simulink model "Forward_model_V4"  (R2018a)
settings: Solver=ode1  StartTime=0.0  StopTime=30  FixedStep=0.001  RelTol=1e-3
InitFcn:
  | Main
values from neighbouring files (symbols this model uses):
  tra_01 = tra_01'    [tra.m]
  tra_02 = tra_02'    [tra.m]
  tra_03 = tra_03'    [tra.m]
  tra_04 = tra_04'    [tra.m]
  tra_05 = tra_05'    [tra.m]
  tra_06 = tra_06'    [tra.m]
undefined symbols (not defined in the file or in its folder): DiscIntNeverNeededParam
libraries: simulink x2
settings Model: Creator=yuxi  LastModifiedBy=yuxi
settings SolverCC: AlgebraicLoopSolver=LineSearch

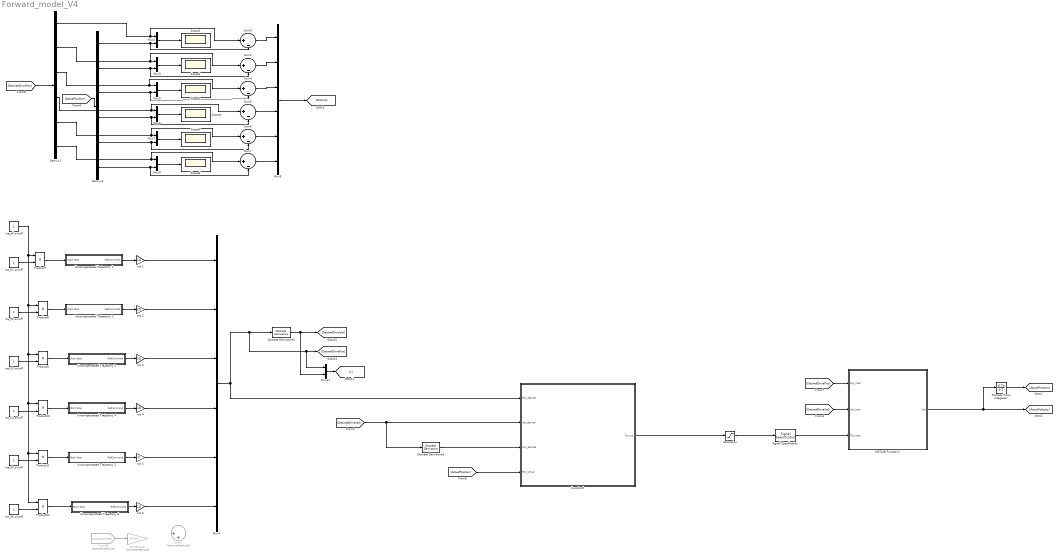
== system Forward_model_V4 ==
  " Function5" : MATLAB Function  TreatAsAtomicUnit=on
  Act J6 pos2 : Gain  Commented=on  Gain=0.025
  Demux1 : Demux  Outputs=6
  Demux4 : Demux  Outputs=6
  Discrete Derivative2 : simulink/Discrete/Discrete Derivative  gainval=1.0  ICPrevScaledInput=0.0  InputProcessing=Inherited  OutMin=[]  OutMax=[]  OutDataType=fixdt(1, 16)  OutScaling=2^-10  DoSatur=off
  Discrete Derivative3 : simulink/Discrete/Discrete Derivative  gainval=1.0  ICPrevScaledInput=0.0  InputProcessing=Inherited  OutMin=[]  OutMax=[]  OutDataType=fixdt(1, 16)  OutScaling=2^-10  DoSatur=off
  Discrete-Time Integrator : DiscreteIntegrator  SampleTime=-1  ICPrevOutput=DiscIntNeverNeededParam  ICPrevScaledInput=DiscIntNeverNeededParam
  From31 : From  Commented=on  GotoTag=ActualPosition5
  MATLAB Function2 : MATLAB Function  TreatAsAtomicUnit=on
  Mux{2..3,5..8,11} (7 alike) : Mux  Inputs=2
  Mux4 : Mux  Inputs=6
  Mux9 : Mux  Inputs=6
  Product{7..12} (6 alike) : Product  RndMeth=Zero
  Saturation : Saturate  UpperLimit=6  LowerLimit=-6
  Scope{1..6} (6 alike) : Scope
  Signal Specification : SignalSpecification  Dimensions=6
  Sum1 : Sum  Commented=on  Inputs=|++
  Sum{2..7} (6 alike) : Sum  Inputs=|+-
  Uncompensated Trajectory 1 : Subsystem
  Uncompensated Trajectory 2 : Subsystem
  Uncompensated Trajectory 3 : Subsystem
  Uncompensated Trajectory 4 : Subsystem
  Uncompensated Trajectory 5 : Subsystem
  Uncompensated Trajectory 6 : Subsystem
  tra 1 : Gain  Gain=10
  tra 2 : Gain  Gain=10
  "tra 3 " : Gain  Gain=10
  "tra 4 " : Gain  Gain=10
  "tra 5 " : Gain  Gain=0
  "tra 6 " : Gain  Gain=10
  tra_01 on/off : Constant
  tra_02 on/off : Constant
  tra_03 on/off : Constant
  tra_04 on/off : Constant
  tra_05 on/off : Constant
  tra_06 on/off : Constant
  tra_all on/off : Constant
  wires:
  [DesiredDrivePos] -> Demux1/1
  [ActualPosition] -> Demux4/1
  Uncompensated Trajectory 2/1(RefCommand) -> tra 2/1
  Uncompensated Trajectory 4/1(RefCommand) -> "tra 4 "/1
  tra_06 on/off/1 -> Product12/2
  Uncompensated Trajectory 1/1(RefCommand) -> tra 1/1
  From31/1 -> Act J6 pos2/1
  tra_02 on/off/1 -> Product8/2
  Product12/1 -> Uncompensated Trajectory 6/1(Start-Stop)
  Product9/1 -> Uncompensated Trajectory 3/1(Start-Stop)
  tra_03 on/off/1 -> Product9/2
  Product11/1 -> Uncompensated Trajectory 5/1(Start-Stop)
  Product10/1 -> Uncompensated Trajectory 4/1(Start-Stop)
  Product7/1 -> Uncompensated Trajectory 1/1(Start-Stop)
  Uncompensated Trajectory 3/1(RefCommand) -> "tra 3 "/1
  tra_04 on/off/1 -> Product10/2
  Uncompensated Trajectory 5/1(RefCommand) -> "tra 5 "/1
  tra_05 on/off/1 -> Product11/2
  Product8/1 -> Uncompensated Trajectory 2/1(Start-Stop)
  Uncompensated Trajectory 6/1(RefCommand) -> "tra 6 "/1
  tra_all on/off/1 -> Product9/1, Product10/1, Product11/1, Product12/1, Product8/1, Product7/1
  tra_01 on/off/1 -> Product7/2
  Discrete-Time Integrator/1 -> [ActualPosition]
  [DesiredDrivePos] -> MATLAB Function2/1(Pos_input)
  [DesiredDriveVel] -> MATLAB Function2/2(Vel_input)
  Demux4/1 -> Sum3/2, Mux2/2
  Demux1/1 -> Sum3/1, Mux2/1
  Demux4/2 -> Sum2/2, Mux3/2
  Demux1/2 -> Sum2/1, Mux3/1
  Demux4/4 -> Sum5/2, Mux6/2
  Demux1/4 -> Sum5/1, Mux6/1
  Demux4/5 -> Sum6/2, Mux7/2
  Demux1/5 -> Sum6/1, Mux7/1
  Demux4/6 -> Sum7/2, Mux8/2
  Demux1/6 -> Sum7/1, Mux8/1
  tra 1/1 -> Mux4/1
  tra 2/1 -> Mux4/2
  "tra 3 "/1 -> Mux4/3
  "tra 4 "/1 -> Mux4/4
  "tra 5 "/1 -> Mux4/5
  "tra 6 "/1 -> Mux4/6
  Mux2/1 -> Scope1/1
  Mux3/1 -> Scope2/1
  Mux5/1 -> Scope3/1
  Mux6/1 -> Scope4/1
  Mux7/1 -> Scope5/1
  Mux8/1 -> Scope6/1
  [DesiredDriveVel] -> Discrete Derivative3/1, " Function5"/2(Vel_desired)
  Discrete Derivative3/1 -> " Function5"/3(Acc_desired)
  Demux1/3 -> Sum4/1, Mux5/1
  Demux4/3 -> Sum4/2, Mux5/2
  Sum6/1 -> Mux9/5
  Sum7/1 -> Mux9/6
  Sum4/1 -> Mux9/3
  Sum2/1 -> Mux9/2
  Sum3/1 -> Mux9/1
  Mux9/1 -> [Disturb]
  Sum5/1 -> Mux9/4
  MATLAB Function2/1(Vel) -> [ActualVelosity], Discrete-Time Integrator/1
  Saturation/1 -> Signal Specification/1
  Signal Specification/1 -> MATLAB Function2/3(Tor_input)
  Mux4/1 -> [DesiredDrivePos], Mux11/1, Discrete Derivative2/1, " Function5"/1(Pos_desired)
  Discrete Derivative2/1 -> [DesiredDriveVel], Mux11/2
  Mux11/1 -> [y]
  " Function5"/1(Tor_out) -> Saturation/1
  [ActualPosition] -> " Function5"/4(Pos_Actual)

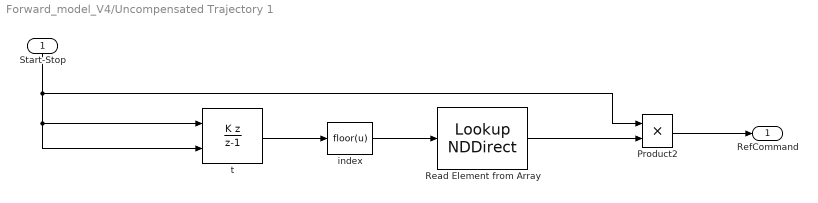
== system Forward_model_V4/Uncompensated Trajectory 1 ==
  Start-Stop : Inport
  Product2 : Product  RndMeth=Zero
  Read Element from Array : LookupNDDirect  NumberOfTableDimensions=1  Table=tra_01
  index : Fcn  Expr=floor(u)
  t : DiscreteIntegrator  IntegratorMethod=Accumulation: Backward Euler  ExternalReset=rising  SampleTime=-1  ICPrevOutput=DiscIntNeverNeededParam  ICPrevScaledInput=DiscIntNeverNeededParam
  RefCommand : Outport
  wires:
  Read Element from Array/1 -> Product2/2
  t/1 -> index/1
  Product2/1 -> RefCommand/1
  Start-Stop/1 -> Product2/1, t/1, t/2
  index/1 -> Read Element from Array/1

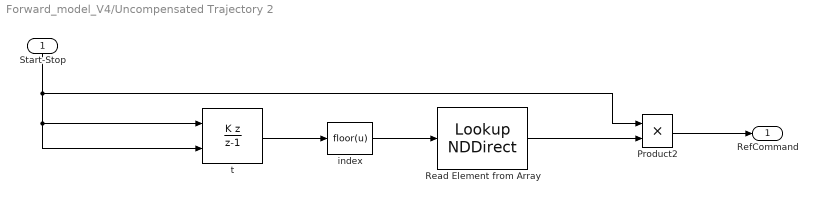
== system Forward_model_V4/Uncompensated Trajectory 2 ==
  Start-Stop : Inport
  Product2 : Product  RndMeth=Zero
  Read Element from Array : LookupNDDirect  NumberOfTableDimensions=1  Table=tra_02
  index : Fcn  Expr=floor(u)
  t : DiscreteIntegrator  IntegratorMethod=Accumulation: Backward Euler  ExternalReset=rising  SampleTime=-1  ICPrevOutput=DiscIntNeverNeededParam  ICPrevScaledInput=DiscIntNeverNeededParam
  RefCommand : Outport
  wires:
  index/1 -> Read Element from Array/1
  Start-Stop/1 -> t/2, t/1, Product2/1
  Product2/1 -> RefCommand/1
  t/1 -> index/1
  Read Element from Array/1 -> Product2/2

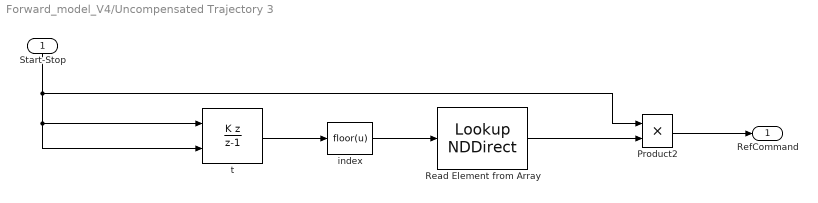
== system Forward_model_V4/Uncompensated Trajectory 3 ==
  Start-Stop : Inport
  Product2 : Product  RndMeth=Zero
  Read Element from Array : LookupNDDirect  NumberOfTableDimensions=1  Table=tra_03
  index : Fcn  Expr=floor(u)
  t : DiscreteIntegrator  IntegratorMethod=Accumulation: Backward Euler  ExternalReset=rising  SampleTime=-1  ICPrevOutput=DiscIntNeverNeededParam  ICPrevScaledInput=DiscIntNeverNeededParam
  RefCommand : Outport
  wires:
  Read Element from Array/1 -> Product2/2
  t/1 -> index/1
  Product2/1 -> RefCommand/1
  Start-Stop/1 -> Product2/1, t/1, t/2
  index/1 -> Read Element from Array/1

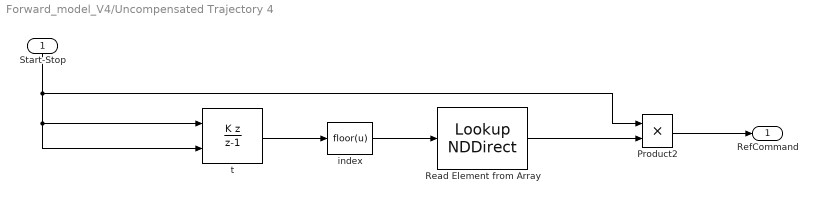
== system Forward_model_V4/Uncompensated Trajectory 4 ==
  Start-Stop : Inport
  Product2 : Product  RndMeth=Zero
  Read Element from Array : LookupNDDirect  NumberOfTableDimensions=1  Table=tra_04
  index : Fcn  Expr=floor(u)
  t : DiscreteIntegrator  IntegratorMethod=Accumulation: Backward Euler  ExternalReset=rising  SampleTime=-1  ICPrevOutput=DiscIntNeverNeededParam  ICPrevScaledInput=DiscIntNeverNeededParam
  RefCommand : Outport
  wires:
  Read Element from Array/1 -> Product2/2
  t/1 -> index/1
  Product2/1 -> RefCommand/1
  Start-Stop/1 -> Product2/1, t/1, t/2
  index/1 -> Read Element from Array/1

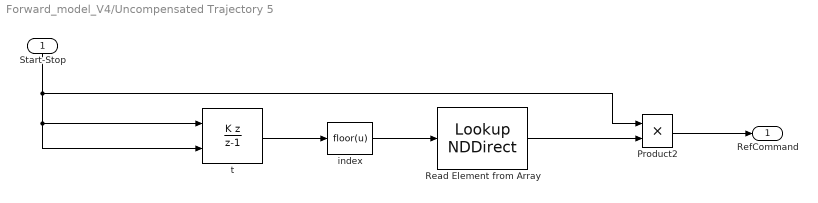
== system Forward_model_V4/Uncompensated Trajectory 5 ==
  Start-Stop : Inport
  Product2 : Product  RndMeth=Zero
  Read Element from Array : LookupNDDirect  NumberOfTableDimensions=1  Table=tra_05
  index : Fcn  Expr=floor(u)
  t : DiscreteIntegrator  IntegratorMethod=Accumulation: Backward Euler  ExternalReset=rising  SampleTime=-1  ICPrevOutput=DiscIntNeverNeededParam  ICPrevScaledInput=DiscIntNeverNeededParam
  RefCommand : Outport
  wires:
  Read Element from Array/1 -> Product2/2
  t/1 -> index/1
  Product2/1 -> RefCommand/1
  Start-Stop/1 -> Product2/1, t/1, t/2
  index/1 -> Read Element from Array/1

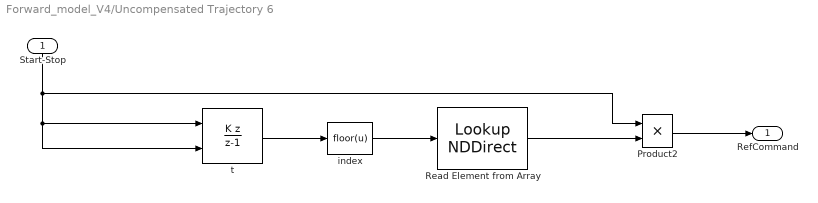
== system Forward_model_V4/Uncompensated Trajectory 6 ==
  Start-Stop : Inport
  Product2 : Product  RndMeth=Zero
  Read Element from Array : LookupNDDirect  NumberOfTableDimensions=1  Table=tra_06
  index : Fcn  Expr=floor(u)
  t : DiscreteIntegrator  IntegratorMethod=Accumulation: Backward Euler  ExternalReset=rising  SampleTime=-1  ICPrevOutput=DiscIntNeverNeededParam  ICPrevScaledInput=DiscIntNeverNeededParam
  RefCommand : Outport
  wires:
  index/1 -> Read Element from Array/1
  Start-Stop/1 -> t/2, t/1, Product2/1
  Product2/1 -> RefCommand/1
  t/1 -> index/1
  Read Element from Array/1 -> Product2/2

== matlab function Forward_model_V4/MATLAB Function2 ==
  data: Pos_input input; Vel_input input; Tor_input input; Vel output; Ts parameter
% Input -- jnt_val: 3x6 -> Joint angles, velocities and accelerations of 6 actuated joints
% [
%   ang_1, ang_2, ang_3, ang_4, ang_5, ang_6;
%   vel_1, vel_2, vel_3, vel_4, vel_5, vel_6;
%   acc_1, acc_2, acc_3, acc_4, acc_5, acc_6;
% ]
% Output -- torques: 6x1 -> For 6 joints
% Time required: 0.25ms
% function [Pos, Vel, Acc] = Robot(ActualPos, ActualVel, Tor)

% This is the forward model of Julun robot, it can be used in simulation
% The author is YuXi

% Pos_input = rand(1,6);
% Vel_input = rand(1,6);
% ActualAcc = zeros(1,6);
% Tor_input = rand(6,1);


function Vel = Robot_model(Pos_input, Vel_input, Tor_input, Ts)

% download the position commands of each joint
Pos_joint1 = Pos_input(1);
Pos_joint2 = Pos_input(2);
Pos_joint3 = Pos_input(3);
Pos_joint4 = Pos_input(4);
Pos_joint5 = Pos_input(5);
Pos_joint6 = Pos_input(6);
Pos_commands = [Pos_joint1 Pos_joint2 Pos_joint3 Pos_joint4 Pos_joint5 Pos_joint6];

% download the velocity commands of each joint
Vel_joint1 = Vel_input(1);
Vel_joint2 = Vel_input(2);
Vel_joint3 = Vel_input(3);
Vel_joint4 = Vel_input(4);
Vel_joint5 = Vel_input(5);
Vel_joint6 = Vel_input(6);
Vel_commands = [Vel_joint1 Vel_joint2 Vel_joint3 Vel_joint4 Vel_joint5 Vel_joint6];

% downlaod the torque informations of each joint
Tor_joint1 = Tor_input(1);
Tor_joint2 = Tor_input(2);
Tor_joint3 = Tor_input(3);
Tor_joint4 = Tor_input(4);
Tor_joint5 = Tor_input(5);
Tor_joint6 = Tor_input(6);
Tor = [Tor_joint1 Tor_joint2 Tor_joint3 Tor_joint4 Tor_joint5 Tor_joint6]';

%% compute the Cdq+Gq

DH = [0, 0, 0, 0; 0, 0.19, pi/2, pi/2; 0, 0.65, 0, 0; 0.73, 0.192, pi/2, 0; 0, 0, pi/2, 0; 0, 0, -pi/2, 0];
iVector = [0,0,0,0,0.844903,0;-0.324345,-0.075914,-0.051391,-0.042523,0.740601,0;-0.091039,0.053809,0.006962,-0.031913,0.049886,0;-0.009236,-0.006692,-0.011727,-0.000768,0.020729,0;-0.004762,0.002377,-0.001658,0.003359,0.000719,0;-0.005854,-0.004165,-0.005599,0.002253,0.001373,0];
mCenter = [0,0.327776,0.067582,-0.004515,0.003987,0.000929;0,0.021804,-0.089291,0.002001,0.00702,-0.001923;0,0,0,0,0,0];
Ia = [0.259947,-0.014791,0.040481,0.013916];
% Fs = [0.372305,0.494409,0.409654,0.063411,0.32759,0.197599];
% Fv = [1.610821,1.074123,0.624158,0.264797,0.327863,0.311985];
% Ia = [0 0 0 0];
Fs = [0 0 0 0 0 0];
Fv = [0 0 0 0 0 0];

iMatrix=zeros(3,3,6);
for i = 1 : 6
    iMatrix(:, :, i) = [iVector(i, 1), iVector(i, 2), iVector(i, 3); iVector(i, 2), iVector(i, 6), iVector(i, 4); iVector(i, 3), iVector(i, 4), iVector(i, 5)];
end   
    
acc_defined = zeros(1,6);       % Set the acceleration to 0, and then compute the torque_*
tor = zeros(6, 1);
rot=zeros(3,3,6);
omega=zeros(3,6);
domega=zeros(3,6);
accer=zeros(3,6);
cforce=zeros(3,6);
force=zeros(3,6);
torque=zeros(3,6);

qval = Pos_commands(1, :);
dqval = Vel_commands(1, :);
ddqval = acc_defined(1, :);
theta = DH(:, 4)' + qval;
pos = [DH(:, 2)'; -(DH(:, 1).*sin(DH(:, 3)))'; (DH(:, 1).*cos(DH(:, 3)))'];

for i = 1 : 6
    rot(:, :, i) = [cos(theta(i)), cos(DH(i, 3))*sin(theta(i)), sin(DH(i, 3))*sin(theta(i)); -sin(theta(i)), cos(DH(i, 3))*cos(theta(i)), sin(DH(i, 3))*cos(theta(i)); 0, -sin(DH(i, 3)), cos(DH(i, 3))];
end

i = 0;
omega_0 = zeros(3, 1);
domega_0 = zeros(3, 1);
accer_0 = [0; 0; 9.80665];
i = 1;
omega(:, i) = [0; 0; dqval(i)];
domega(:, i) = [0; 0; ddqval(i)];
accer(:, i) = rot(:, :, i) * accer_0;
cforce(:, i) = cross(domega(:, i), mCenter(:, i)) + cross(omega(:, i), cross(omega(:, i), mCenter(:, i)));

for i = 2 : 6
    omega(:, i) = rot(:, :, i) * omega(:, i - 1) + [0; 0; dqval(i)];
    domega(:, i) = rot(:, :, i) * domega(:, i - 1) + cross(rot(:, :, i)*omega(:, i - 1), [0; 0; dqval(i)]) + [0; 0; ddqval(i)];
    accer(:, i) = rot(:, :, i) * (accer(:, i - 1) + (cross(domega(:, i - 1), pos(:, i))) + (cross(omega(:, i - 1), cross(omega(:, i - 1), pos(:, i)))));
    cforce(:, i) = cross(domega(:, i), mCenter(:, i)) + cross(omega(:, i), cross(omega(:, i), mCenter(:, i)));
end

i = 6;
force(:, i) = cforce(:, i);
torque(:, i) = iMatrix(:, :, i) * domega(:, i) + cross(omega(:, i), iMatrix(:, :, i)*omega(:, i)) + cross(mCenter(:, i), accer(:, i));
tor(i) = torque(3, i);

for i = 5 : -1 : 1
    force(:, i) = cforce(:, i) + rot(:, :, i+1)' * force(:, i+1);
    torque(:, i) = iMatrix(:, :, i) * domega(:, i) + cross(omega(:, i), iMatrix(:, :, i)*omega(:, i)) + cross(mCenter(:, i), accer(:, i)) + rot(:, :, i+1)' * torque(:, i+1) + cross(pos(:, i+1), rot(:, :, i+1)'*force(:, i+1));
    tor(i) = torque(3, i);
end

tor = tor + (Fs.*sign(dqval))' + (Fv.*dqval)' + ([0, 0, Ia].*ddqval)';

% tor = tor + ([0, 0, Ia].*ddqval)';
Tor_delta = Tor - tor;

%% compute the M(q)

Eye_matrix = eye(6);
tor = zeros(6, 1);
rot=zeros(3,3,6);
omega=zeros(3,6);
domega=zeros(3,6);
accer=zeros(3,6);
cforce=zeros(3,6);
force=zeros(3,6);
torque=zeros(3,6);
H = zeros(6,6);
Vel_commands2 = zeros(1,6);                % Set the velocity to 0

for j = 1:6
    acc_defined2 = Eye_matrix(:,j)';       % Set each colume to unit vector
    qval = Pos_commands(1, :);
    dqval = Vel_commands2(1, :);
    ddqval = acc_defined2(1, :);
    theta = DH(:, 4)' + qval;
    pos = [DH(:, 2)'; -(DH(:, 1).*sin(DH(:, 3)))'; (DH(:, 1).*cos(DH(:, 3)))'];
    
    for i = 1 : 6
        rot(:, :, i) = [cos(theta(i)), cos(DH(i, 3))*sin(theta(i)), sin(DH(i, 3))*sin(theta(i)); -sin(theta(i)), cos(DH(i, 3))*cos(theta(i)), sin(DH(i, 3))*cos(theta(i)); 0, -sin(DH(i, 3)), cos(DH(i, 3))];
    end
    
    i = 0;
    omega_0 = zeros(3, 1);
    domega_0 = zeros(3, 1);
    accer_0 = [0; 0; 0];        % 重力加速度设置为0
    i = 1;
    omega(:, i) = [0; 0; dqval(i)];
    domega(:, i) = [0; 0; ddqval(i)];
    accer(:, i) = rot(:, :, i) * accer_0;
    cforce(:, i) = cross(domega(:, i), mCenter(:, i)) + cross(omega(:, i), cross(omega(:, i), mCenter(:, i)));
    cforce(:, i) = cross(domega(:, i), mCenter(:, i)) + cross(omega(:, i), cross(omega(:, i), mCenter(:, i)));
    
    for i = 2 : 6
        omega(:, i) = rot(:, :, i) * omega(:, i - 1) + [0; 0; dqval(i)];
        domega(:, i) = rot(:, :, i) * domega(:, i - 1) + cross(rot(:, :, i)*omega(:, i - 1), [0; 0; dqval(i)]) + [0; 0; ddqval(i)];
        accer(:, i) = rot(:, :, i) * (accer(:, i - 1) + (cross(domega(:, i - 1), pos(:, i))) + (cross(omega(:, i - 1), cross(omega(:, i - 1), pos(:, i)))));
        cforce(:, i) = cross(domega(:, i), mCenter(:, i)) + cross(omega(:, i), cross(omega(:, i), mCenter(:, i)));
    end
    
    i = 6;
    force(:, i) = cforce(:, i);
    torque(:, i) = iMatrix(:, :, i) * domega(:, i) + cross(omega(:, i), iMatrix(:, :, i)*omega(:, i)) + cross(mCenter(:, i), accer(:, i));
    tor(i) = torque(3, i);
    
    for i = 5 : -1 : 1
        force(:, i) = cforce(:, i) + rot(:, :, i+1)' * force(:, i+1);
        torque(:, i) = iMatrix(:, :, i) * domega(:, i) + cross(omega(:, i), iMatrix(:, :, i)*omega(:, i)) + cross(mCenter(:, i), accer(:, i)) + rot(:, :, i+1)' * torque(:, i+1) + cross(pos(:, i+1), rot(:, :, i+1)'*force(:, i+1));
        tor(i) = torque(3, i);
    end
    
%     H(:,j) = tor + (Fs.*sign(dqval))' + (Fv.*dqval)';
    H(:,j) = tor;
    
end

%% compute the ddq

% Acc = (inv(H) * Tor_delta)';
Acc = (inv(H + diag([0, 0, Ia])) * Tor_delta)';
Vel = (Vel_commands + Acc * Ts)';

% Pos = (Pos_commands + Vel_commands * Ts + 0.5 * Acc * (Ts).^2)';    
          
end

== matlab function Forward_model_V4/ Function5 ==
  data: Tor_out output; Pos_desired input; Vel_desired input; Acc_desired input; Pos_Actual input

% function Vel = Robot_LQR(Pos_input, Vel_input, Tor_input, Ts)

% Input -- jnt_val: 3x6 -> Joint angles, velocities and accelerations of 6 actuated joints
% [
%   ang_1, ang_2, ang_3, ang_4, ang_5, ang_6;
%   vel_1, vel_2, vel_3, vel_4, vel_5, vel_6;
%   acc_1, acc_2, acc_3, acc_4, acc_5, acc_6;
% ]
% Output -- torques: 6x1 -> For 6 joints
% Time required: 0.25ms
% function [Pos, Vel, Acc] = Robot(ActualPos, ActualVel, Tor)

% This is the forward model of Julun robot, it can be used in simulation
% The author is YuXi

% function [Tor_out, A, B, H, D] = Robot_LQR_X(Pos_desired, Vel_desired, Acc_desired, Actual_Esti)
function Tor_out  = Robot_LQR_X(Pos_desired, Vel_desired, Acc_desired, Pos_Actual)


% Pos_desired = rand(1,6);
% Pos_actual = Pos_desired;
% Vel_desired = rand(1,6);
% Vel_actual = Vel_desired;
% Acc_actual = rand(1,6);

coder.extrinsic('lqr');

% download the desired position commands of each joint
Pos_j1 = Pos_desired(1);
Pos_j2 = Pos_desired(2);
Pos_j3 = Pos_desired(3);
Pos_j4 = Pos_desired(4);
Pos_j5 = Pos_desired(5);
Pos_j6 = Pos_desired(6);
Pos_Desired = [Pos_j1 Pos_j2 Pos_j3 Pos_j4 Pos_j5 Pos_j6];
% Pos_Desired = [Pos_j1 Pos_j2 Pos_j3 Pos_j4 Pos_j5 Pos_j6 zeros(1,6)];

% download the desired position commands of each joint
Vel_j1 = Vel_desired(1);
Vel_j2 = Vel_desired(2);
Vel_j3 = Vel_desired(3);
Vel_j4 = Vel_desired(4);
Vel_j5 = Vel_desired(5);
Vel_j6 = Vel_desired(6);
Vel_Desired = [Vel_j1 Vel_j2 Vel_j3 Vel_j4 Vel_j5 Vel_j6];

% download the actual acceleration commands of each joint
Acc_joint1 = Acc_desired(1);
Acc_joint2 = Acc_desired(2);
Acc_joint3 = Acc_desired(3);
Acc_joint4 = Acc_desired(4);
Acc_joint5 = Acc_desired(5);
Acc_joint6 = Acc_desired(6);
Acc_Desired = [Acc_joint1 Acc_joint2 Acc_joint3 Acc_joint4 Acc_joint5 Acc_joint6];

%% the parameters

DH = [0, 0, 0, 0; 0, 0.19, pi/2, pi/2; 0, 0.65, 0, 0; 0.73, 0.192, pi/2, 0; 0, 0, pi/2, 0; 0, 0, -pi/2, 0];
iVector = [0,0,0,0,0.844903,0;-0.324345,-0.075914,-0.051391,-0.042523,0.740601,0;-0.091039,0.053809,0.006962,-0.031913,0.049886,0;-0.009236,-0.006692,-0.011727,-0.000768,0.020729,0;-0.004762,0.002377,-0.001658,0.003359,0.000719,0;-0.005854,-0.004165,-0.005599,0.002253,0.001373,0];
mCenter = [0,0.327776,0.067582,-0.004515,0.003987,0.000929;0,0.021804,-0.089291,0.002001,0.00702,-0.001923;0,0,0,0,0,0];
Ia = [0.259947,-0.014791,0.040481,0.013916];
% Fs = [0.372305,0.494409,0.409654,0.063411,0.32759,0.197599];
% Fv = [1.610821,1.074123,0.624158,0.264797,0.327863,0.311985];
% Ia = [0 0 0 0];
Fs = [0 0 0 0 0 0];
Fv = [0 0 0 0 0 0];

iMatrix=zeros(3,3,6);
for i = 1 : 6
    iMatrix(:, :, i) = [iVector(i, 1), iVector(i, 2), iVector(i, 3); iVector(i, 2), iVector(i, 6), iVector(i, 4); iVector(i, 3), iVector(i, 4), iVector(i, 5)];
end

%% the Tor_all

tor = zeros(6, 1);
rot=zeros(3,3,6);
omega=zeros(3,6);
domega=zeros(3,6);
accer=zeros(3,6);
cforce=zeros(3,6);
force=zeros(3,6);
torque=zeros(3,6);

qval = Pos_Desired(1, :);
dqval = Vel_Desired(1, :);
ddqval = Acc_Desired(1, :);
theta = DH(:, 4)' + qval;
pos = [DH(:, 2)'; -(DH(:, 1).*sin(DH(:, 3)))'; (DH(:, 1).*cos(DH(:, 3)))'];
for i = 1 : 6
    rot(:, :, i) = [cos(theta(i)), cos(DH(i, 3))*sin(theta(i)), sin(DH(i, 3))*sin(theta(i)); -sin(theta(i)), cos(DH(i, 3))*cos(theta(i)), sin(DH(i, 3))*cos(theta(i)); 0, -sin(DH(i, 3)), cos(DH(i, 3))];
end
i = 0;
omega_0 = zeros(3, 1);
domega_0 = zeros(3, 1);
accer_0 = [0; 0; 9.80665];
i = 1;
omega(:, i) = [0; 0; dqval(i)];
domega(:, i) = [0; 0; ddqval(i)];
accer(:, i) = rot(:, :, i) * accer_0;
cforce(:, i) = cross(domega(:, i), mCenter(:, i)) + cross(omega(:, i), cross(omega(:, i), mCenter(:, i)));
for i = 2 : 6
    omega(:, i) = rot(:, :, i) * omega(:, i - 1) + [0; 0; dqval(i)];
    domega(:, i) = rot(:, :, i) * domega(:, i - 1) + cross(rot(:, :, i)*omega(:, i - 1), [0; 0; dqval(i)]) + [0; 0; ddqval(i)];
    accer(:, i) = rot(:, :, i) * (accer(:, i - 1) + (cross(domega(:, i - 1), pos(:, i))) + (cross(omega(:, i - 1), cross(omega(:, i - 1), pos(:, i)))));
    cforce(:, i) = cross(domega(:, i), mCenter(:, i)) + cross(omega(:, i), cross(omega(:, i), mCenter(:, i)));
end
i = 6;
force(:, i) = cforce(:, i);
torque(:, i) = iMatrix(:, :, i) * domega(:, i) + cross(omega(:, i), iMatrix(:, :, i)*omega(:, i)) + cross(mCenter(:, i), accer(:, i));
tor(i) = torque(3, i);
for i = 5 : -1 : 1
    force(:, i) = cforce(:, i) + rot(:, :, i+1)' * force(:, i+1);
    torque(:, i) = iMatrix(:, :, i) * domega(:, i) + cross(omega(:, i), iMatrix(:, :, i)*omega(:, i)) + cross(mCenter(:, i), accer(:, i)) + rot(:, :, i+1)' * torque(:, i+1) + cross(pos(:, i+1), rot(:, :, i+1)'*force(:, i+1));
    tor(i) = torque(3, i);
end
Tor = tor;
Tor_d = (Fs.*sign(Vel_Desired))' + (Fv.*Vel_Desired)'  + ([0, 0, Ia].*ddqval)';
% Tor_d = (Fv.*Vel_Desired)'  + ([0, 0, Ia].*ddqval)';

%% compute the Hq.  The matrix of M(q)

Eye_matrix = eye(6);
tor = zeros(6, 1);
rot=zeros(3,3,6);
omega=zeros(3,6);
domega=zeros(3,6);
accer=zeros(3,6);
cforce=zeros(3,6);
force=zeros(3,6);
torque=zeros(3,6);
M = zeros(6,6);
Vel_commands2 = zeros(1,6);                % Set the velocity to 0    

for j = 1:6
    acc_defined2 = Eye_matrix(:,j)';       % Set each colume to unit vector
    qval = Pos_Desired(1, :);
    dqval = Vel_commands2(1, :);
    ddqval = acc_defined2(1, :);
    theta = DH(:, 4)' + qval;
    pos = [DH(:, 2)'; -(DH(:, 1).*sin(DH(:, 3)))'; (DH(:, 1).*cos(DH(:, 3)))'];
    
    for i = 1 : 6
        rot(:, :, i) = [cos(theta(i)), cos(DH(i, 3))*sin(theta(i)), sin(DH(i, 3))*sin(theta(i)); -sin(theta(i)), cos(DH(i, 3))*cos(theta(i)), sin(DH(i, 3))*cos(theta(i)); 0, -sin(DH(i, 3)), cos(DH(i, 3))];
    end
    
    i = 0;
    omega_0 = zeros(3, 1);
    domega_0 = zeros(3, 1);
    accer_0 = [0; 0; 0];        % 重力加速度设置为0
    i = 1;
    omega(:, i) = [0; 0; dqval(i)];
    domega(:, i) = [0; 0; ddqval(i)];
    accer(:, i) = rot(:, :, i) * accer_0;
    cforce(:, i) = cross(domega(:, i), mCenter(:, i)) + cross(omega(:, i), cross(omega(:, i), mCenter(:, i)));
    cforce(:, i) = cross(domega(:, i), mCenter(:, i)) + cross(omega(:, i), cross(omega(:, i), mCenter(:, i)));
    
    for i = 2 : 6
        omega(:, i) = rot(:, :, i) * omega(:, i - 1) + [0; 0; dqval(i)];
        domega(:, i) = rot(:, :, i) * domega(:, i - 1) + cross(rot(:, :, i)*omega(:, i - 1), [0; 0; dqval(i)]) + [0; 0; ddqval(i)];
        accer(:, i) = rot(:, :, i) * (accer(:, i - 1) + (cross(domega(:, i - 1), pos(:, i))) + (cross(omega(:, i - 1), cross(omega(:, i - 1), pos(:, i)))));
        cforce(:, i) = cross(domega(:, i), mCenter(:, i)) + cross(omega(:, i), cross(omega(:, i), mCenter(:, i)));
    end
    
    i = 6;
    force(:, i) = cforce(:, i);
    torque(:, i) = iMatrix(:, :, i) * domega(:, i) + cross(omega(:, i), iMatrix(:, :, i)*omega(:, i)) + cross(mCenter(:, i), accer(:, i));
    tor(i) = torque(3, i);
    
    for i = 5 : -1 : 1
        force(:, i) = cforce(:, i) + rot(:, :, i+1)' * force(:, i+1);
        torque(:, i) = iMatrix(:, :, i) * domega(:, i) + cross(omega(:, i), iMatrix(:, :, i)*omega(:, i)) + cross(mCenter(:, i), accer(:, i)) + rot(:, :, i+1)' * torque(:, i+1) + cross(pos(:, i+1), rot(:, :, i+1)'*force(:, i+1));
        tor(i) = torque(3, i);
    end
    
%     M(:,j) = tor + (Fs.*sign(dqval))' + (Fv.*dqval)';   
    M(:,j) = tor;    

end

Mddq = M * Acc_Desired';
    
    
%% compute the C(q,dq) /  G(q)

tor = zeros(6, 1);
rot=zeros(3,3,6);
omega=zeros(3,6);
domega=zeros(3,6);
accer=zeros(3,6);
cforce=zeros(3,6);
force=zeros(3,6);
torque=zeros(3,6);
% acc_defined3 = zeros(1,6);

qval = Pos_Desired(1, :);
dqval = Vel_Desired(1, :);
ddqval = Acc_Desired(1, :);
theta = DH(:, 4)' + qval;
pos = [DH(:, 2)'; -(DH(:, 1).*sin(DH(:, 3)))'; (DH(:, 1).*cos(DH(:, 3)))'];
for i = 1 : 6
    rot(:, :, i) = [cos(theta(i)), cos(DH(i, 3))*sin(theta(i)), sin(DH(i, 3))*sin(theta(i)); -sin(theta(i)), cos(DH(i, 3))*cos(theta(i)), sin(DH(i, 3))*cos(theta(i)); 0, -sin(DH(i, 3)), cos(DH(i, 3))];
end
i = 0;
omega_0 = zeros(3, 1);
domega_0 = zeros(3, 1);
accer_0 = [0; 0; 0];
i = 1;
omega(:, i) = [0; 0; dqval(i)];
domega(:, i) = [0; 0; ddqval(i)];
accer(:, i) = rot(:, :, i) * accer_0;
cforce(:, i) = cross(domega(:, i), mCenter(:, i)) + cross(omega(:, i), cross(omega(:, i), mCenter(:, i)));
for i = 2 : 6
    omega(:, i) = rot(:, :, i) * omega(:, i - 1) + [0; 0; dqval(i)];
    domega(:, i) = rot(:, :, i) * domega(:, i - 1) + cross(rot(:, :, i)*omega(:, i - 1), [0; 0; dqval(i)]) + [0; 0; ddqval(i)];
    accer(:, i) = rot(:, :, i) * (accer(:, i - 1) + (cross(domega(:, i - 1), pos(:, i))) + (cross(omega(:, i - 1), cross(omega(:, i - 1), pos(:, i)))));
    cforce(:, i) = cross(domega(:, i), mCenter(:, i)) + cross(omega(:, i), cross(omega(:, i), mCenter(:, i)));
end
i = 6;
force(:, i) = cforce(:, i);
torque(:, i) = iMatrix(:, :, i) * domega(:, i) + cross(omega(:, i), iMatrix(:, :, i)*omega(:, i)) + cross(mCenter(:, i), accer(:, i));
tor(i) = torque(3, i);
for i = 5 : -1 : 1
    force(:, i) = cforce(:, i) + rot(:, :, i+1)' * force(:, i+1);
    torque(:, i) = iMatrix(:, :, i) * domega(:, i) + cross(omega(:, i), iMatrix(:, :, i)*omega(:, i)) + cross(mCenter(:, i), accer(:, i)) + rot(:, :, i+1)' * torque(:, i+1) + cross(pos(:, i+1), rot(:, :, i+1)'*force(:, i+1));
    tor(i) = torque(3, i);
end

Tor_0 = tor;
% Tor_0 = tor + (Fs.*sign(Vel_Desired))' + (Fv.*Vel_Desired)';
G = (Tor - Tor_0) * pinv(Pos_Desired');
C = (Tor_0 - Mddq) * pinv(Vel_Desired');
   
%% compute the coffiencient of matrix A,B,C

% Tor_out = Mddq + C * Vel_Desired' + G * Pos_Desired';
% Tor_out = Mddq + C * Vel_Desired' + G * Pos_Desired' + Tor_d;

% Tor_out = Mddq;

% delta_tor = Tor - Tor_out;

A = [zeros(6,6) eye(6);      
     -pinv(M)*G -pinv(M)*C];       % A: (12,12)
B = [zeros(6,6);
     pinv(M)];                     % B: (12,6)
H = [eye(6) zeros(6); zeros(6,12)];                   % C: (12,12)
D = zeros(12,6);

%% LQR

% Q_temp = [0.9 0.8 0.01 0.5 0.01 0.01 20 20 0.5 150 0 0];   % 缺省值
Q_temp = [0.9 0.8 0.01 10 0.01 0.01 20 20 0.5 1.0 0 0];   % 缺省值

% Q_temp = [1 1 1 1 1 1 10 10 10 10 10 10];   % 缺省值

Q = diag(Q_temp);
% R_temp = [50 50 500 100000000 500000 500000];    % 缺省值
R_temp = [50 50 500 100000 500 50000000];    % 缺省值

% R_temp = [1 1 1 1 1 1];    % 缺省值

R = diag(R_temp);
K = zeros(6,12);
K = lqr(A, B, Q, R);
% P = pinv(B')*R*K;

X = Pos_Actual;

Tor_out = -K * [X;0;0;0;0;0;0];
end
